simulink model "Project"  (R2023b)
settings: Solver=VariableStepAuto  StartTime=0.0  StopTime=10.0  RelTol=1e-3
values from neighbouring files (symbols this model uses):
  Cn = 2.3 * 3600    (= 8280)    [Project_Run.m]
  I = 2.3    [Project_Run.m]
  OCV = Data(:,2)    [Project_Run.m]
  R_Discharge = Data(:,4)    [Project_Run.m]
  SOC = Data(:,1)    [Project_Run.m]
settings Model: Creator=Lenovo  LastModifiedBy=Lenovo

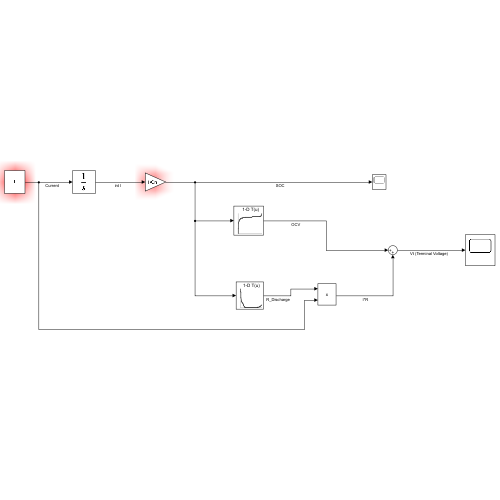
[thumbnail: Simulink's stored preview of the top-level diagram]
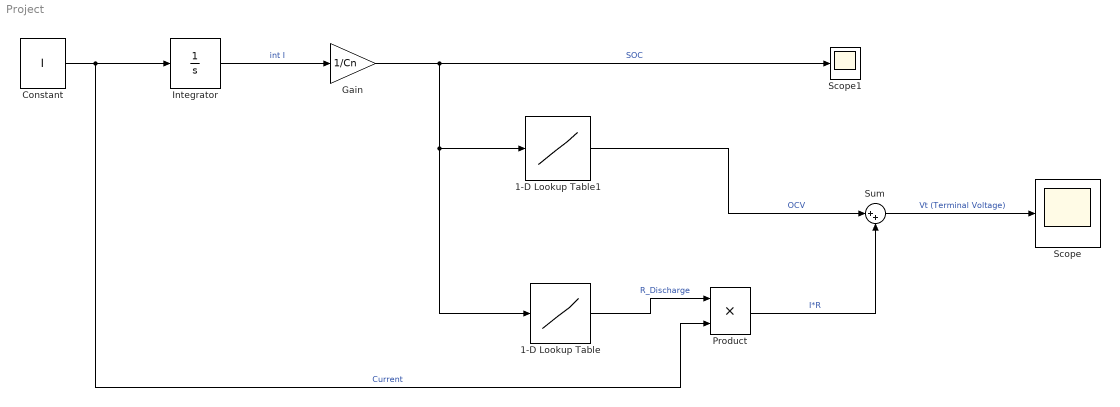
== system Project ==
  1-D Lookup Table : Lookup_n-D  NumberOfTableDimensions=1  BreakpointsForDimension1=SOC  Table=R_Discharge  InternalRulePriority=Speed  RndMeth=Simplest
  1-D Lookup Table1 : Lookup_n-D  NumberOfTableDimensions=1  BreakpointsForDimension1=SOC  Table=OCV  InternalRulePriority=Speed  RndMeth=Simplest
  Constant : Constant  Value=I
  Gain : Gain  Gain=1/Cn
  Integrator : Integrator
  Product : Product
  Scope : Scope
  Scope1 : Scope
  Sum : Sum  Inputs=|++
  wires:
  Constant/1 -> Product/2, Integrator/1  "Current"
  Integrator/1 -> Gain/1  "int I"
  Gain/1 -> Scope1/1, 1-D Lookup Table/1, 1-D Lookup Table1/1  "SOC"
  1-D Lookup Table/1 -> Product/1  "R_Discharge"
  1-D Lookup Table1/1 -> Sum/1  "OCV"
  Product/1 -> Sum/2  "I*R"
  Sum/1 -> Scope/1  "Vt (Terminal Voltage)"
